simulink model "fz5_8"  (R2014a)
settings: Solver=ode45  StartTime=0.0  StopTime=5  MaxStep=0.001  RelTol=1e-3
undefined symbols (not defined in the file or in its folder): magnitude
libraries: commanapbnd3 x3, dsparch4 x2, commchan3 x1, dspstat3 x1, commrandsrc2 x1
settings Model: Creator=tzb  LastModifiedBy=tzb

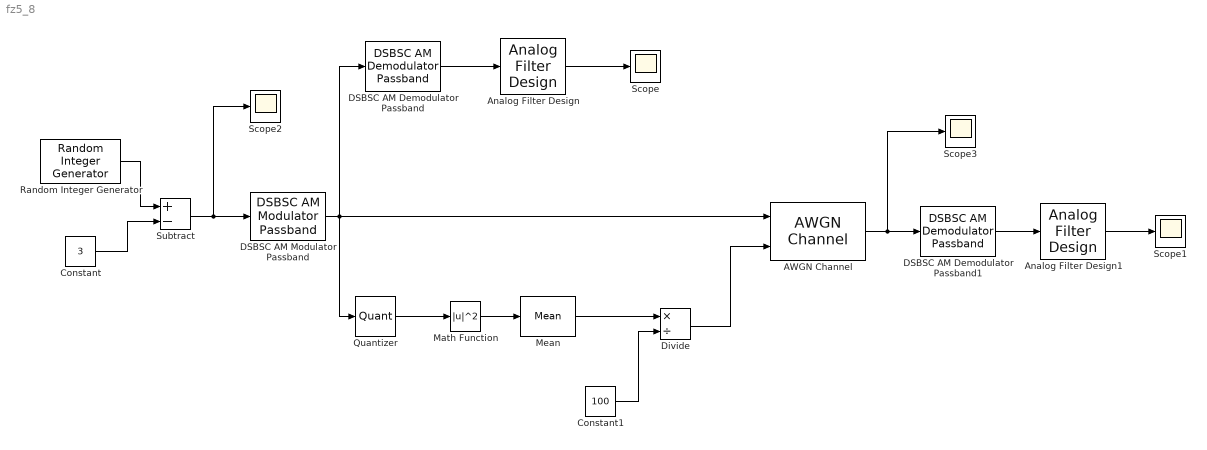
== system fz5_8 ==
  AWGN Channel : commchan3/AWGN Channel  InputProcessing=Columns as channels (frame based)  seed=67  noiseMode=Variance from port  EbNodB=10  EsNodB=10  SNRdB=10  bitsPerSym=1  Ps=1  Tsym=1  variance=1
  Analog Filter Design : dsparch4/Analog Filter Design  method=Butterworth  filttype=Lowpass  N=8  Wlo=30  Whi=80  Rp=2  Rs=40
  Analog Filter Design1 : dsparch4/Analog Filter Design  method=Butterworth  filttype=Lowpass  N=8  Wlo=30  Whi=80  Rp=2  Rs=40
  Constant : Constant  Value=3
  Constant1 : Constant  Value=100
  DSBSC AM Demodulator Passband : commanapbnd3/DSBSC AM Demodulator Passband  Fc=300  Ph=0  method=Butterworth  n=4  cf=300  Rp=0.1  Rs=50
  DSBSC AM Demodulator Passband1 : commanapbnd3/DSBSC AM Demodulator Passband  Fc=300  Ph=0  method=Butterworth  n=4  cf=300  Rp=0.1  Rs=50
  DSBSC AM Modulator Passband : commanapbnd3/DSBSC AM Modulator Passband  Fc=300  Ph=0
  Divide : Product  Inputs=*/
  Math Function : Math  Operator=magnitude^2  SaturateOnIntegerOverflow=on
  Mean : dspstat3/Mean  run=on  reset_popup=None  InputProcessing=Columns as channels (frame based)  directionMode=Each column  dimension=1  treatSBRowAsCol=on  roiEnable=off  roiType=Rectangles  roiPortion=Entire ROI  roiOutput=Individual statistics for each ROI  roiFlag=off  outputDataTypeStr=Inherit: Same as accumulator  outputLastDataTypeStr=Inherit: Same as accumulator  outputMin=[]  outputMax=[]  roundingMode=Floor  overflowMode=off
  Quantizer : Quantizer  QuantizationInterval=0.001  LinearizeAsGain=off  SampleTime=0.001
  Random Integer Generator : commrandsrc2/Random Integer Generator  mul=7  seed=37  Ts=1/10  frameBased=off  sampPerFrame=1  orient=off  outDataType=double
  Scope{,1..3} (4 alike) : Scope
      Scope2 settings: SaveName=ScopeData2
      Scope3 settings: SaveName=ScopeData3
  Subtract : Sum  Inputs=+-
  wires:
  Random Integer Generator/1 -> Subtract/1
  Constant/1 -> Subtract/2
  Subtract/1 -> Scope2/1, DSBSC AM Modulator Passband/1
  Quantizer/1 -> Math Function/1
  Math Function/1 -> Mean/1
  Mean/1 -> Divide/1
  Constant1/1 -> Divide/2
  Divide/1 -> AWGN Channel/2
  DSBSC AM Demodulator Passband1/1 -> Analog Filter Design1/1
  Analog Filter Design1/1 -> Scope1/1
  AWGN Channel/1 -> Scope3/1, DSBSC AM Demodulator Passband1/1
  DSBSC AM Modulator Passband/1 -> Quantizer/1, DSBSC AM Demodulator Passband/1, AWGN Channel/1
  DSBSC AM Demodulator Passband/1 -> Analog Filter Design/1
  Analog Filter Design/1 -> Scope/1
